simulink model "simul"  (R2024a)
settings: Solver=VariableStepAuto  StartTime=0.0  StopTime=100  FixedStep=1e-4  MaxStep=1e-3  RelTol=1e-3
undefined symbols (not defined in the file or in its folder): DiscIntNeverNeededParam
libraries: matrix_library x3
settings Model: Creator=Ych_0  LastModifiedBy=Ych_0

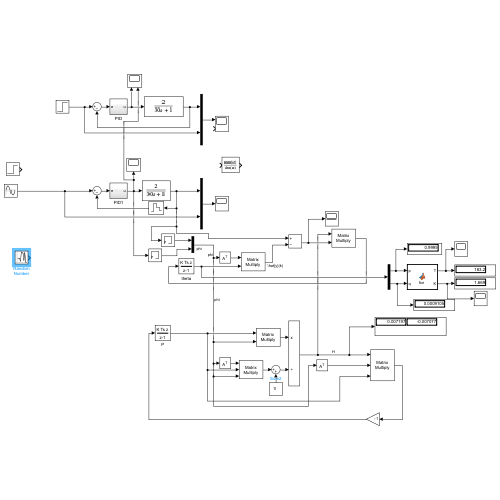
[thumbnail: Simulink's stored preview of the top-level diagram]
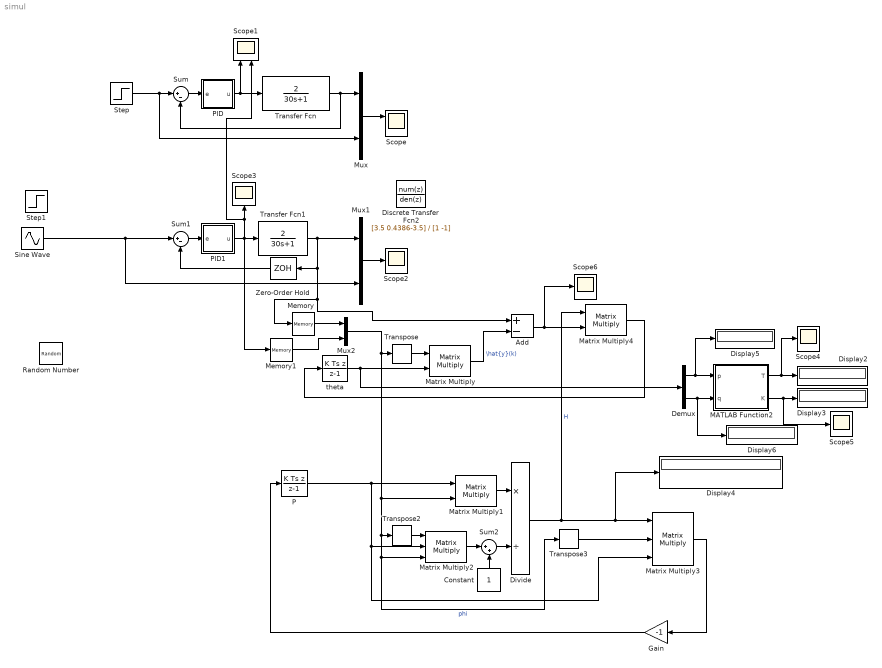
== system simul ==
  Add : Sum  Inputs=+-
  Constant : Constant
  Demux : Demux  Outputs=2
  Discrete Transfer Fcn2 : DiscreteTransferFcn  Numerator=[3.5 0.4386-3.5]  Denominator=[1 -1]
  Display{2..6} (5 alike) : Display
  Divide : Product  Inputs=*/
  Gain : Gain  Gain=-1
  MATLAB Function2 : MATLAB Function  TreatAsAtomicUnit=on
  Matrix Multiply : Product  Multiplication=Matrix(*)
  Matrix Multiply1 : Product  Multiplication=Matrix(*)
  Matrix Multiply2 : Product  Inputs=3  Multiplication=Matrix(*)
  Matrix Multiply3 : Product  Inputs=3  Multiplication=Matrix(*)
  Matrix Multiply4 : Product  Multiplication=Matrix(*)
  Memory : Memory
  Memory1 : Memory
  Mux : Mux  Inputs=2
  Mux1 : Mux  Inputs=2
  Mux2 : Mux  Inputs=2
  P : DiscreteIntegrator  IntegratorMethod=Integration: Backward Euler  InitialCondition=100*[1 0;0 1]  SampleTime=0.01  ICPrevOutput=DiscIntNeverNeededParam  ICPrevScaledInput=DiscIntNeverNeededParam
  PID : Subsystem
  PID1 : Subsystem
  Random Number : RandomNumber  Mean=30  Variance=10  Seed=123  SampleTime=1
  Scope : Scope  NumInputPorts=2
  Scope1 : Scope  NumInputPorts=2
  Scope{2..6} (5 alike) : Scope
  Sine Wave : Sin  Frequency=0.05  SampleTime=0
  Step : Step  Time=0  After=60  SampleTime=0
  Step1 : Step  Time=0  After=60  SampleTime=0
  Sum : Sum  Inputs=|+-
  Sum1 : Sum  Inputs=|+-
  Sum2 : Sum  Inputs=|++
  Transfer Fcn : TransferFcn  Numerator=2  Denominator=[30 1]
  Transfer Fcn1 : TransferFcn  Numerator=2  Denominator=[30 1]
  Transpose : matrix_library/Transpose
  Transpose2 : matrix_library/Transpose
  Transpose3 : matrix_library/Transpose
  Zero-Order Hold : ZeroOrderHold  SampleTime=0.1
  theta : DiscreteIntegrator  IntegratorMethod=Integration: Backward Euler  InitialCondition=[0.5;0.5]  SampleTime=0.01  ICPrevOutput=DiscIntNeverNeededParam  ICPrevScaledInput=DiscIntNeverNeededParam
  wires:
  Step/1 -> Mux/2, Sum/1
  Transfer Fcn/1 -> Mux/1, Sum/2
  Sum/1 -> PID/1(e)
  PID/1(u) -> Transfer Fcn/1, Scope1/1
  Mux/1 -> Scope/1
  Mux1/1 -> Scope2/1
  Sum1/1 -> PID1/1(e)
  Sine Wave/1 -> Sum1/1, Mux1/2
  Zero-Order Hold/1 -> Sum1/2
  Matrix Multiply/1 -> Add/2  "\\hat{y}(k)"
  theta/1 -> Demux/1, Matrix Multiply/2
  Transpose/1 -> Matrix Multiply/1
  Add/1 -> Scope6/1, Matrix Multiply4/2
  Matrix Multiply1/1 -> Divide/1
  Divide/1 -> Matrix Multiply4/1, Display4/1, Matrix Multiply3/1  "H"
  Matrix Multiply2/1 -> Sum2/1
  Sum2/1 -> Divide/2
  Constant/1 -> Sum2/2
  Transpose2/1 -> Matrix Multiply2/1
  Transpose3/1 -> Matrix Multiply3/2
  Matrix Multiply3/1 -> Gain/1
  Mux2/1 -> Matrix Multiply1/2, Transpose3/1, Matrix Multiply2/3, Transpose2/1, Transpose/1  "phi"
  Gain/1 -> P/1
  Matrix Multiply4/1 -> theta/1
  MATLAB Function2/1(T) -> Scope4/1, Display2/1
  Demux/1 -> Display5/1, MATLAB Function2/1(p)
  Demux/2 -> Display6/1, MATLAB Function2/2(q)
  MATLAB Function2/2(K) -> Scope5/1, Display3/1
  P/1 -> Matrix Multiply1/1, Matrix Multiply2/2, Matrix Multiply3/3
  PID1/1(u) -> Memory1/1, Transfer Fcn1/1, Scope1/2, Scope3/1
  Transfer Fcn1/1 -> Mux1/1, Memory/1, Add/1, Zero-Order Hold/1
  Memory/1 -> Mux2/1
  Memory1/1 -> Mux2/2

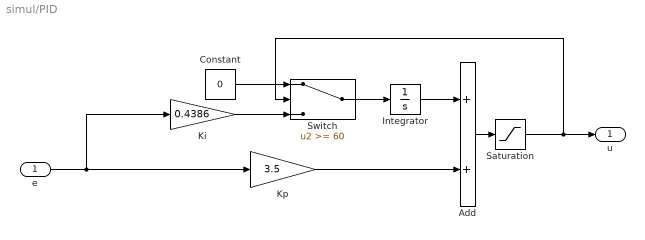
== system simul/PID ==
  e : Inport
  Add : Sum
  Constant : Constant  Value=0
  Integrator : Integrator
  Ki : Gain  Gain=0.4386
  Kp : Gain  Gain=3.5
  Saturation : Saturate  UpperLimit=60  LowerLimit=0
  Switch : Switch  Threshold=60  SaturateOnIntegerOverflow=off  InputSameDT=off
  u : Outport
  wires:
  Kp/1 -> Add/2
  e/1 -> Kp/1, Ki/1
  Integrator/1 -> Add/1
  Ki/1 -> Switch/3
  Constant/1 -> Switch/1
  Add/1 -> Saturation/1
  Switch/1 -> Integrator/1
  Saturation/1 -> Switch/2, u/1

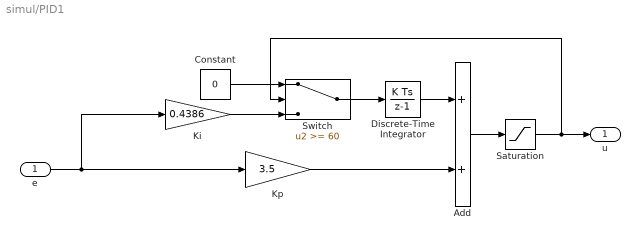
== system simul/PID1 ==
  e : Inport
  Add : Sum
  Constant : Constant  Value=0
  Discrete-Time Integrator : DiscreteIntegrator  SampleTime=0.1  ICPrevOutput=DiscIntNeverNeededParam  ICPrevScaledInput=DiscIntNeverNeededParam
  Ki : Gain  Gain=0.4386
  Kp : Gain  Gain=3.5
  Saturation : Saturate  UpperLimit=60  LowerLimit=0
  Switch : Switch  Threshold=60  SaturateOnIntegerOverflow=off  InputSameDT=off
  u : Outport
  wires:
  Kp/1 -> Add/2
  e/1 -> Kp/1, Ki/1
  Discrete-Time Integrator/1 -> Add/1
  Ki/1 -> Switch/3
  Constant/1 -> Switch/1
  Add/1 -> Saturation/1
  Switch/1 -> Discrete-Time Integrator/1
  Saturation/1 -> Switch/2, u/1

== matlab function simul/MATLAB Function2 ==
  data: p input; T output; q input; K output
function [T,K] = fcn(p,q)
Ts = 0.1;
T = -Ts/log(p);
K = q/(1-p);
